simulink model "test"  (Simulink 7.8)
settings: Solver=ode45  StartTime=0.0  StopTime=1  RelTol=1e-3
undefined symbols (not defined in the file): Fs, get, i, sided, Two
libraries: commsink2 x6, commrandsrc2 x1, dspsnks4 x1, commfilt2 x1
settings Model: Creator=myownreality  LastModifiedBy=myownreality

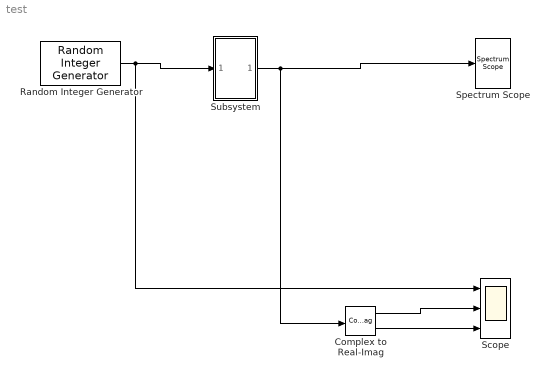
== system test ==
  Complex to Real-Imag : ComplexToRealImag
  Random Integer Generator : commrandsrc2/Random Integer Generator  mul=16  seed=37  Ts=1/9600  frameBased=off  sampPerFrame=1  orient=off  outDataType=double
  Scope : Scope  NumInputPorts=3
      settings: YMin=-0~-2~-2  YMax=15~2~2
  Spectrum Scope : dspsnks4/Spectrum Scope  ScopeProperties=on  Domain=Frequency  HorizSpan=1  UseBuffer=on  BufferSize=1024  Overlap=0  TreatMby1Signals=One channel  inpFftLenInherit=on  FFTlength=1024  numAvg=2  DisplayProperties=off  AxisGrid=on  Memory=off  FrameNumber=on  AxisLegend=off  AxisZoom=off  OpenScopeAtSimStart=on  OpenScopeImmediately=off  FigPos=get(0,'defaultfigureposition')  AxisProperties=off  XUnits=Hertz  XRange=Two-sided ((-Fs/2...Fs/2])  XDisplay=0  InheritXIncr=on  XIncr=1.0  XLabel=Samples  XLimit=User-defined  YUnits=dBW/Hertz  XMax=38400  XMin=-38400  YLabel=Magnitude-squared, dB  LineProperties=off  wintypeSpecScope=Hann  RsSpecScope=50  betaSpecScope=5  winsampSpecScope=Periodic  XAxisParamsVer=6.9  isFrameUpgraded=on
      settings: YMin=-139.206  YMax=-25.9287
  Subsystem : Subsystem
  wires:
  Random Integer Generator/1 -> Subsystem/1(In1), Scope/1
  Subsystem/1(Out1) -> Spectrum Scope/1, Complex to Real-Imag/1
  Complex to Real-Imag/1 -> Scope/2
  Complex to Real-Imag/2 -> Scope/3

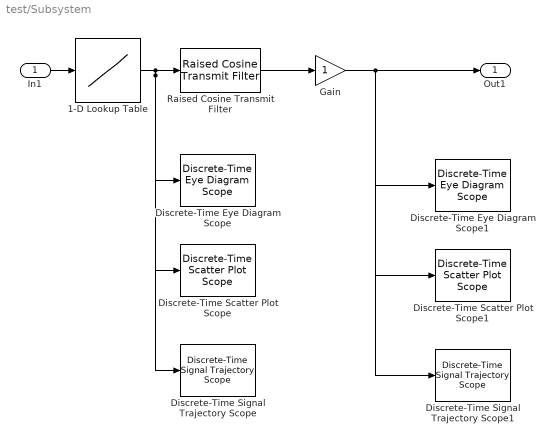
== system test/Subsystem ==
  In1 : Inport
  1-D Lookup Table : Lookup_n-D  NumberOfTableDimensions=1  BreakpointsForDimension1=[0:15]  Table=[ -3+3*i,-3+1*i,-3-3*i,-3-1*i,-1+3*i,-1+1*i,-1-3*i,-1-1*i,+3+3*i,+3+1*i,+3-3*i,+3-1*i,+1+3*i,+1+1*i,+1-3*i,+1-1*i ]  RndMeth=Simplest  InputSameDT=on
  Discrete-Time Eye Diagram Scope : commsink2/Discrete-Time Eye Diagram Scope  Tag=EyeDiagram  sampPerSymb=8  offsetEye=0  symbPerTrace=1  numTraces=200  numNewFrames=40  LineStyles=-  LineColors=b  dupPoints=on  fading=on  render=on  AxisGrid=on  yMin=-3.15  yMax=3.15  inphaseLabel=In-phase Amplitude  quadratureLabel=Quadrature Amplitude  openScopeAtSimStart=on  dispDiagram=In-phase and Quadrature  FrameNumber=off  FigPos=get(0,'defaultfigureposition');  figTitle=Eye Diagram  block_type_=eye  numLinesMax=8
  Discrete-Time Eye Diagram Scope1 : commsink2/Discrete-Time Eye Diagram Scope  Tag=EyeDiagram  sampPerSymb=8  offsetEye=0  symbPerTrace=1  numTraces=200  numNewFrames=40  LineStyles=-  LineColors=b  dupPoints=on  fading=on  render=on  AxisGrid=on  yMin=-4.71751458931147  yMax=4.20326962933122  inphaseLabel=In-phase Amplitude  quadratureLabel=Quadrature Amplitude  openScopeAtSimStart=on  dispDiagram=In-phase and Quadrature  FrameNumber=off  FigPos=get(0,'defaultfigureposition');  figTitle=Eye Diagram  block_type_=eye  numLinesMax=8
  Discrete-Time Scatter Plot Scope : commsink2/Discrete-Time Scatter Plot Scope  Tag=ScatterPlot  sampPerSymb=1  offsetEye=0  numTraces=200  numNewFrames=40  LineMarkers=.  LineColors=b  fading=on  render=on  AxisGrid=on  xMin=-3.3  xMax=3.315  yMin=-3.3  yMax=3.315  inphaseLabel=In-phase Amplitude  quadratureLabel=Quadrature Amplitude  openScopeAtSimStart=on  FrameNumber=off  FigPos=get(0,'defaultfigureposition');  figTitle=Scatter Plot  numLinesMax=8  block_type_=scatter
  Discrete-Time Scatter Plot Scope1 : commsink2/Discrete-Time Scatter Plot Scope  Tag=ScatterPlot  sampPerSymb=1  offsetEye=0  numTraces=2000  numNewFrames=40  LineMarkers=.  LineColors=b  fading=on  render=on  AxisGrid=on  xMin=-1.73154938436308  xMax=1.72426887203724  yMin=-1.73439270633481  yMax=1.72142555006551  inphaseLabel=In-phase Amplitude  quadratureLabel=Quadrature Amplitude  openScopeAtSimStart=on  FrameNumber=off  FigPos=get(0,'defaultfigureposition');  figTitle=Scatter Plot  numLinesMax=8  block_type_=scatter
  Discrete-Time Signal Trajectory Scope : commsink2/Discrete-Time Signal Trajectory Scope  Tag=SignalTrajectory  sampPerSymb=8  offsetEye=0  numTraces=200  numNewFrames=40  LineStyles=-  LineColors=b  fading=on  render=on  AxisGrid=on  xMin=-3.3  xMax=3.315  yMin=-3.3  yMax=3.315  inphaseLabel=In-phase Amplitude  quadratureLabel=Quadrature Amplitude  openScopeAtSimStart=on  FrameNumber=off  FigPos=get(0,'defaultfigureposition');  figTitle=Signal Trajectory  numLinesMax=8  block_type_=xy
  Discrete-Time Signal Trajectory Scope1 : commsink2/Discrete-Time Signal Trajectory Scope  Tag=SignalTrajectory  sampPerSymb=8  offsetEye=0  numTraces=200  numNewFrames=40  LineStyles=-  LineColors=b  fading=on  render=on  AxisGrid=on  xMin=-3.3  xMax=3.315  yMin=-3.3  yMax=3.315  inphaseLabel=In-phase Amplitude  quadratureLabel=Quadrature Amplitude  openScopeAtSimStart=on  FrameNumber=off  FigPos=get(0,'defaultfigureposition');  figTitle=Signal Trajectory  numLinesMax=8  block_type_=xy
  Gain : Gain
  Raised Cosine Transmit Filter : commfilt2/Raised Cosine Transmit Filter  filtType=Square root  D=5  R=1  sampMode=Mute  saveAsFlag=0  N=8  framing=Allow multirate processing  checkGain=Normalized  filterGain=1  checkCoeff=off  variableName=rcTxFilt  launchFVT=off  roundingMode=Floor  overflowMode=off
  Out1 : Outport
  wires:
  In1/1 -> 1-D Lookup Table/1
  1-D Lookup Table/1 -> Raised Cosine Transmit Filter/1, Discrete-Time Scatter Plot Scope/1, Discrete-Time Eye Diagram Scope/1, Discrete-Time Signal Trajectory Scope/1
  Raised Cosine Transmit Filter/1 -> Gain/1
  Gain/1 -> Out1/1, Discrete-Time Eye Diagram Scope1/1, Discrete-Time Scatter Plot Scope1/1, Discrete-Time Signal Trajectory Scope1/1
